simulink subsystem "battery_pack"  (R2021a)
settings: Solver=VariableStepAuto  StartTime=0.0  StopTime=10.0  RelTol=1e-3
values from neighbouring files (symbols this model uses):
  AmbientTemperature = 25 + 273.15    (= 298.15)    [battery_ws.m]
undefined symbols (not defined in the file or in its folder): BusbarRes, CellSeriesRes
libraries: fl_lib x11
settings Model: Creator=Carlo Edoardo  LastModifiedBy=Carlo Edoardo

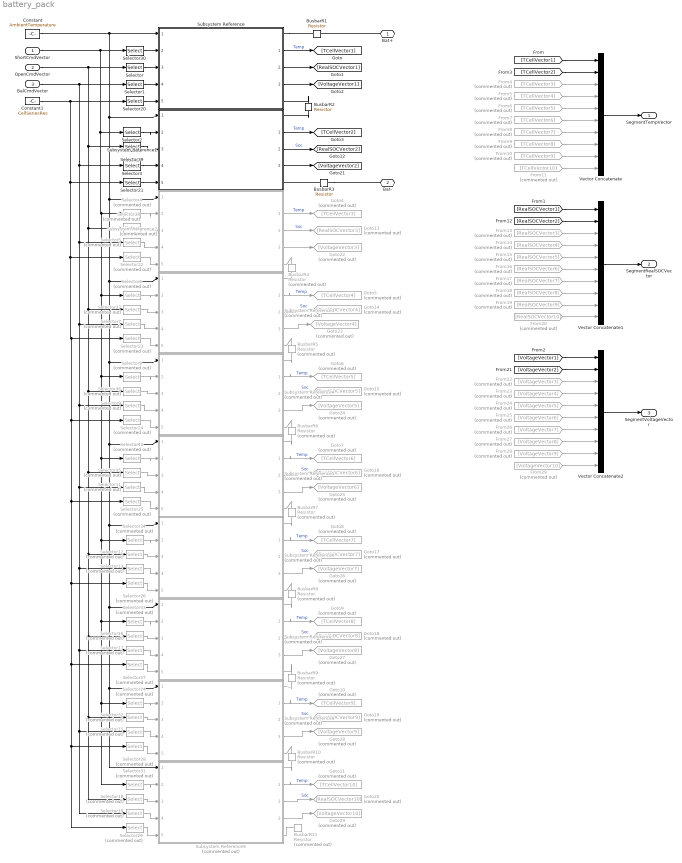
== system battery_pack ==
  ShortCmdVector : Inport
  OpenCmdVector : Inport  Port=2
  BalCmdVector : Inport  Port=3
  BusbarR1 : fl_lib/Electrical/Electrical Elements/Resistor  R=BusbarRes(1) Ohm  i_specify=off  i_priority=None  i=0 A  i_nominal_specify=off  i_nominal_unit=A  i_nominal_value=1  v_specify=off  v_priority=None  v=0 V  v_nominal_specify=off  v_nominal_unit=V  v_nominal_value=1
  BusbarR10 : fl_lib/Electrical/Electrical Elements/Resistor  Commented=on  R=BusbarRes(10) Ohm  i_specify=off  i_priority=None  i=0 A  i_nominal_specify=off  i_nominal_unit=A  i_nominal_value=1  v_specify=off  v_priority=None  v=0 V  v_nominal_specify=off  v_nominal_unit=V  v_nominal_value=1
  BusbarR11 : fl_lib/Electrical/Electrical Elements/Resistor  Commented=on  R=BusbarRes(11) Ohm  i_specify=off  i_priority=None  i=0 A  i_nominal_specify=off  i_nominal_unit=A  i_nominal_value=1  v_specify=off  v_priority=None  v=0 V  v_nominal_specify=off  v_nominal_unit=V  v_nominal_value=1
  BusbarR2 : fl_lib/Electrical/Electrical Elements/Resistor  R=BusbarRes(2) Ohm  i_specify=off  i_priority=None  i=0 A  i_nominal_specify=off  i_nominal_unit=A  i_nominal_value=1  v_specify=off  v_priority=None  v=0 V  v_nominal_specify=off  v_nominal_unit=V  v_nominal_value=1
  BusbarR3 : fl_lib/Electrical/Electrical Elements/Resistor  R=BusbarRes(3) Ohm  i_specify=off  i_priority=None  i=0 A  i_nominal_specify=off  i_nominal_unit=A  i_nominal_value=1  v_specify=off  v_priority=None  v=0 V  v_nominal_specify=off  v_nominal_unit=V  v_nominal_value=1
  BusbarR4 : fl_lib/Electrical/Electrical Elements/Resistor  Commented=on  R=BusbarRes(4) Ohm  i_specify=off  i_priority=None  i=0 A  i_nominal_specify=off  i_nominal_unit=A  i_nominal_value=1  v_specify=off  v_priority=None  v=0 V  v_nominal_specify=off  v_nominal_unit=V  v_nominal_value=1
  BusbarR5 : fl_lib/Electrical/Electrical Elements/Resistor  Commented=on  R=BusbarRes(5) Ohm  i_specify=off  i_priority=None  i=0 A  i_nominal_specify=off  i_nominal_unit=A  i_nominal_value=1  v_specify=off  v_priority=None  v=0 V  v_nominal_specify=off  v_nominal_unit=V  v_nominal_value=1
  BusbarR6 : fl_lib/Electrical/Electrical Elements/Resistor  Commented=on  R=BusbarRes(6) Ohm  i_specify=off  i_priority=None  i=0 A  i_nominal_specify=off  i_nominal_unit=A  i_nominal_value=1  v_specify=off  v_priority=None  v=0 V  v_nominal_specify=off  v_nominal_unit=V  v_nominal_value=1
  BusbarR7 : fl_lib/Electrical/Electrical Elements/Resistor  Commented=on  R=BusbarRes(7) Ohm  i_specify=off  i_priority=None  i=0 A  i_nominal_specify=off  i_nominal_unit=A  i_nominal_value=1  v_specify=off  v_priority=None  v=0 V  v_nominal_specify=off  v_nominal_unit=V  v_nominal_value=1
  BusbarR8 : fl_lib/Electrical/Electrical Elements/Resistor  Commented=on  R=BusbarRes(8) Ohm  i_specify=off  i_priority=None  i=0 A  i_nominal_specify=off  i_nominal_unit=A  i_nominal_value=1  v_specify=off  v_priority=None  v=0 V  v_nominal_specify=off  v_nominal_unit=V  v_nominal_value=1
  BusbarR9 : fl_lib/Electrical/Electrical Elements/Resistor  Commented=on  R=BusbarRes(9) Ohm  i_specify=off  i_priority=None  i=0 A  i_nominal_specify=off  i_nominal_unit=A  i_nominal_value=1  v_specify=off  v_priority=None  v=0 V  v_nominal_specify=off  v_nominal_unit=V  v_nominal_value=1
  Constant : Constant  Value=AmbientTemperature
  Constant1 : Constant  Value=CellSeriesRes
  From10 : From  Commented=on  GotoTag=TCellVector9
  From11 : From  Commented=on  GotoTag=TCellVector10
  From13 : From  Commented=on  GotoTag=RealSOCVector3
  From14 : From  Commented=on  GotoTag=RealSOCVector4
  From15 : From  Commented=on  GotoTag=RealSOCVector5
  From16 : From  Commented=on  GotoTag=RealSOCVector6
  From17 : From  Commented=on  GotoTag=RealSOCVector7
  From18 : From  Commented=on  GotoTag=RealSOCVector8
  From19 : From  Commented=on  GotoTag=RealSOCVector9
  From20 : From  Commented=on  GotoTag=RealSOCVector10
  From22 : From  Commented=on  GotoTag=VoltageVector3
  From23 : From  Commented=on  GotoTag=VoltageVector4
  From24 : From  Commented=on  GotoTag=VoltageVector5
  From25 : From  Commented=on  GotoTag=VoltageVector6
  From26 : From  Commented=on  GotoTag=VoltageVector7
  From27 : From  Commented=on  GotoTag=VoltageVector8
  From28 : From  Commented=on  GotoTag=VoltageVector9
  From29 : From  Commented=on  GotoTag=VoltageVector10
  From4 : From  Commented=on  GotoTag=TCellVector3
  From5 : From  Commented=on  GotoTag=TCellVector4
  From6 : From  Commented=on  GotoTag=TCellVector5
  From7 : From  Commented=on  GotoTag=TCellVector6
  From8 : From  Commented=on  GotoTag=TCellVector7
  From9 : From  Commented=on  GotoTag=TCellVector8
  Goto10 : Goto  Commented=on  GotoTag=TCellVector9
  Goto11 : Goto  Commented=on  GotoTag=TCellVector10
  Goto13 : Goto  Commented=on  GotoTag=RealSOCVector3
  Goto14 : Goto  Commented=on  GotoTag=RealSOCVector4
  Goto15 : Goto  Commented=on  GotoTag=RealSOCVector5
  Goto16 : Goto  Commented=on  GotoTag=RealSOCVector6
  Goto17 : Goto  Commented=on  GotoTag=RealSOCVector7
  Goto18 : Goto  Commented=on  GotoTag=RealSOCVector8
  Goto19 : Goto  Commented=on  GotoTag=RealSOCVector9
  Goto20 : Goto  Commented=on  GotoTag=RealSOCVector10
  Goto22 : Goto  Commented=on  GotoTag=VoltageVector3
  Goto23 : Goto  Commented=on  GotoTag=VoltageVector4
  Goto24 : Goto  Commented=on  GotoTag=VoltageVector5
  Goto25 : Goto  Commented=on  GotoTag=VoltageVector6
  Goto26 : Goto  Commented=on  GotoTag=VoltageVector7
  Goto27 : Goto  Commented=on  GotoTag=VoltageVector8
  Goto28 : Goto  Commented=on  GotoTag=VoltageVector9
  Goto29 : Goto  Commented=on  GotoTag=VoltageVector10
  Goto4 : Goto  Commented=on  GotoTag=TCellVector3
  Goto5 : Goto  Commented=on  GotoTag=TCellVector4
  Goto6 : Goto  Commented=on  GotoTag=TCellVector5
  Goto7 : Goto  Commented=on  GotoTag=TCellVector6
  Goto8 : Goto  Commented=on  GotoTag=TCellVector7
  Goto9 : Goto  Commented=on  GotoTag=TCellVector8
  Selector{,1,20,30} (4 alike) : Selector  InputPortWidth=10  IndexOptions=Index vector (dialog)  Indices=1  OutputSizes=1
  Selector{10..11,25,35} (4 alike) : Selector  Commented=on  InputPortWidth=10  IndexOptions=Index vector (dialog)  Indices=6  OutputSizes=1
  Selector{12..13,26,34} (4 alike) : Selector  Commented=on  InputPortWidth=10  IndexOptions=Index vector (dialog)  Indices=7  OutputSizes=1
  Selector{14..15,28,32} (4 alike) : Selector  Commented=on  InputPortWidth=10  IndexOptions=Index vector (dialog)  Indices=9  OutputSizes=1
  Selector{16..17,27,33} (4 alike) : Selector  Commented=on  InputPortWidth=10  IndexOptions=Index vector (dialog)  Indices=8  OutputSizes=1
  Selector{18..19,29,31} (4 alike) : Selector  Commented=on  InputPortWidth=10  IndexOptions=Index vector (dialog)  Indices=10  OutputSizes=1
  Selector{2..3,21,39} (4 alike) : Selector  InputPortWidth=10  IndexOptions=Index vector (dialog)  Indices=2  OutputSizes=1
  Selector{4..5,22,38} (4 alike) : Selector  Commented=on  InputPortWidth=10  IndexOptions=Index vector (dialog)  Indices=3  OutputSizes=1
  Selector{6..7,23,37} (4 alike) : Selector  Commented=on  InputPortWidth=10  IndexOptions=Index vector (dialog)  Indices=4  OutputSizes=1
  Selector{8..9,24,36} (4 alike) : Selector  Commented=on  InputPortWidth=10  IndexOptions=Index vector (dialog)  Indices=5  OutputSizes=1
  Subsystem Reference : Subsystem  ReferencedSubsystem=battery_module
      settings: PortSchema="{\"entries\":[{\"content\":{\"sides\":[{\"content\":{\"connectorIds\":[\"In1\",\"In2\",\"In3\",\"In4\",\"In5\"]},\"type\":\"ConnectorPlacement.EquallySpacedRectSide\",\"uuid\":\"f42d6b3d-39c7-468b-a9a7-4e5d796eba3b\"},{\"content\":{\"connectorIds\":[\"RConn1\",\"Out1\",\"Out2\",\"Out3\",\"RConn2\"],\"side\":\"RIGHT\"},\"type\":\"ConnectorPlacement.EquallySpacedRectSide\",\"uuid\":\"e762e236-7776-43b9-bd8d-fb7f2716d190\"},{\"content\":{\"connectorIds\":[],\"side\":\"TOP\"},\"type\":\"ConnectorPlacement.EquallySpacedRectSide\",\"uuid\":\"bd0c4b53-2dd2-497f-95b6-77c2ca394183\"}]},\"type\":\"ConnectorPlacement.EquallySpacedConnector\",\"uuid\":\"abacbee7-c859-4f21-9973-420371fecb92\"}],\"packageUris\":[\"http://schema.mathworks.com/mf0/Connector/R2020b\"],\"version\":\"1.0\"}"
  Subsystem Reference1 : Subsystem  ReferencedSubsystem=battery_module
      settings: PortSchema="{\"entries\":[{\"content\":{\"sides\":[{\"content\":{\"connectorIds\":[\"In1\",\"In2\",\"In3\",\"In4\",\"In5\"]},\"type\":\"ConnectorPlacement.EquallySpacedRectSide\",\"uuid\":\"f42d6b3d-39c7-468b-a9a7-4e5d796eba3b\"},{\"content\":{\"connectorIds\":[\"RConn1\",\"Out1\",\"Out2\",\"Out3\",\"RConn2\"],\"side\":\"RIGHT\"},\"type\":\"ConnectorPlacement.EquallySpacedRectSide\",\"uuid\":\"e762e236-7776-43b9-bd8d-fb7f2716d190\"},{\"content\":{\"connectorIds\":[],\"side\":\"TOP\"},\"type\":\"ConnectorPlacement.EquallySpacedRectSide\",\"uuid\":\"bd0c4b53-2dd2-497f-95b6-77c2ca394183\"}]},\"type\":\"ConnectorPlacement.EquallySpacedConnector\",\"uuid\":\"abacbee7-c859-4f21-9973-420371fecb92\"}],\"packageUris\":[\"http://schema.mathworks.com/mf0/Connector/R2020b\"],\"version\":\"1.0\"}"
  Subsystem Reference{2..9} (8 alike) : Subsystem  Commented=on  ReferencedSubsystem=battery_module
      settings: PortSchema="{\"entries\":[{\"content\":{\"sides\":[{\"content\":{\"connectorIds\":[\"In1\",\"In2\",\"In3\",\"In4\",\"In5\"]},\"type\":\"ConnectorPlacement.EquallySpacedRectSide\",\"uuid\":\"f42d6b3d-39c7-468b-a9a7-4e5d796eba3b\"},{\"content\":{\"connectorIds\":[\"RConn1\",\"Out1\",\"Out2\",\"Out3\",\"RConn2\"],\"side\":\"RIGHT\"},\"type\":\"ConnectorPlacement.EquallySpacedRectSide\",\"uuid\":\"e762e236-7776-43b9-bd8d-fb7f2716d190\"},{\"content\":{\"connectorIds\":[],\"side\":\"TOP\"},\"type\":\"ConnectorPlacement.EquallySpacedRectSide\",\"uuid\":\"bd0c4b53-2dd2-497f-95b6-77c2ca394183\"}]},\"type\":\"ConnectorPlacement.EquallySpacedConnector\",\"uuid\":\"abacbee7-c859-4f21-9973-420371fecb92\"}],\"packageUris\":[\"http://schema.mathworks.com/mf0/Connector/R2020b\"],\"version\":\"1.0\"}"
  Vector Concatenate : Concatenate  NumInputs=10
  Vector Concatenate1 : Concatenate  NumInputs=10
  Vector Concatenate2 : Concatenate  NumInputs=10
  Bat+ : PMIOPort  Side=Right
  Bat- : PMIOPort  Port=2  Side=Right
  SegmentTempVector : Outport
  SegmentRealSOCVector : Outport  Port=2
  SegmentVoltageVector : Outport  Port=3
  wires:
  Subsystem Reference8/1 -> Goto10/1  "Temp"
  [VoltageVector1] -> Vector Concatenate2/1
  Selector8/1 -> Subsystem Reference4/2
  Selector22/1 -> Subsystem Reference2/5
  Selector34/1 -> Subsystem Reference6/2
  From22/1 -> Vector Concatenate2/3
  Subsystem Reference8/2 -> Goto19/1  "Soc"
  From27/1 -> Vector Concatenate2/8
  Selector28/1 -> Subsystem Reference8/5
  ShortCmdVector/1 -> Selector30/1, Selector2/1, Selector4/1, Selector6/1, Selector8/1, Selector10/1, Selector34/1, Selector33/1, Selector14/1, Selector31/1
  Subsystem Reference5/2 -> Goto16/1  "Soc"
  Selector17/1 -> Subsystem Reference7/4
  From24/1 -> Vector Concatenate2/5
  Selector13/1 -> Subsystem Reference6/4
  From23/1 -> Vector Concatenate2/4
  From4/1 -> Vector Concatenate/3
  From16/1 -> Vector Concatenate1/6
  Selector6/1 -> Subsystem Reference3/2
  From5/1 -> Vector Concatenate/4
  Selector3/1 -> Subsystem Reference1/4
  From6/1 -> Vector Concatenate/5
  Constant/1 -> Subsystem Reference/1, Subsystem Reference3/1, Subsystem Reference9/1, Subsystem Reference8/1, Subsystem Reference7/1, Subsystem Reference6/1, Subsystem Reference5/1, Subsystem Reference4/1, Subsystem Reference2/1, Subsystem Reference1/1
  [VoltageVector2] -> Vector Concatenate2/2
  Subsystem Reference4/2 -> Goto15/1  "Soc"
  Selector25/1 -> Subsystem Reference5/5
  Selector10/1 -> Subsystem Reference5/2
  Selector35/1 -> Subsystem Reference5/3
  Subsystem Reference9/3 -> Goto29/1
  Subsystem Reference7/2 -> Goto18/1  "Soc"
  Selector24/1 -> Subsystem Reference4/5
  Constant1/1 -> Selector20/1, Selector21/1, Selector22/1, Selector23/1, Selector24/1, Selector25/1, Selector26/1, Selector27/1, Selector28/1, Selector29/1
  Selector37/1 -> Subsystem Reference3/3
  Subsystem Reference5/3 -> Goto25/1
  From29/1 -> Vector Concatenate2/10
  [TCellVector2] -> Vector Concatenate/2
  Subsystem Reference7/1 -> Goto9/1  "Temp"
  BalCmdVector/1 -> Selector1/1, Selector3/1, Selector5/1, Selector7/1, Selector9/1, Selector11/1, Selector13/1, Selector17/1, Selector15/1, Selector19/1
  From25/1 -> Vector Concatenate2/6
  From20/1 -> Vector Concatenate1/10
  Subsystem Reference6/3 -> Goto26/1
  Subsystem Reference4/1 -> Goto6/1  "Temp"
  From28/1 -> Vector Concatenate2/9
  Vector Concatenate2/1 -> SegmentVoltageVector/1
  Subsystem Reference3/1 -> Goto5/1  "Temp"
  Selector31/1 -> Subsystem Reference9/2
  From26/1 -> Vector Concatenate2/7
  Selector26/1 -> Subsystem Reference6/5
  Selector23/1 -> Subsystem Reference3/5
  Selector/1 -> Subsystem Reference/3
  Selector16/1 -> Subsystem Reference7/3
  Selector7/1 -> Subsystem Reference3/4
  From19/1 -> Vector Concatenate1/9
  Selector5/1 -> Subsystem Reference2/4
  Selector4/1 -> Subsystem Reference2/2
  Selector2/1 -> Subsystem Reference1/2
  Selector38/1 -> Subsystem Reference2/3
  Selector39/1 -> Subsystem Reference1/3
  From18/1 -> Vector Concatenate1/8
  Subsystem Reference3/2 -> Goto14/1  "Soc"
  Subsystem Reference/2 -> [RealSOCVector1]
  Subsystem Reference2/1 -> Goto4/1  "Temp"
  OpenCmdVector/1 -> Selector39/1, Selector38/1, Selector37/1, Selector36/1, Selector35/1, Selector12/1, Selector16/1, Selector32/1, Selector18/1, Selector/1
  Vector Concatenate1/1 -> SegmentRealSOCVector/1
  Subsystem Reference5/1 -> Goto7/1  "Temp"
  Subsystem Reference/1 -> [TCellVector1]  "Temp"
  [TCellVector1] -> Vector Concatenate/1
  From11/1 -> Vector Concatenate/10
  From8/1 -> Vector Concatenate/7
  Subsystem Reference/3 -> [VoltageVector1]
  Selector21/1 -> Subsystem Reference1/5
  From10/1 -> Vector Concatenate/9
  Subsystem Reference6/2 -> Goto17/1  "Soc"
  [RealSOCVector1] -> Vector Concatenate1/1
  Selector12/1 -> Subsystem Reference6/3
  From14/1 -> Vector Concatenate1/4
  From13/1 -> Vector Concatenate1/3
  Subsystem Reference2/2 -> Goto13/1  "Soc"
  Subsystem Reference9/2 -> Goto20/1  "Soc"
  Selector11/1 -> Subsystem Reference5/4
  Subsystem Reference1/2 -> [RealSOCVector2]  "Soc"
  From15/1 -> Vector Concatenate1/5
  Subsystem Reference2/3 -> Goto22/1
  From17/1 -> Vector Concatenate1/7
  Subsystem Reference4/3 -> Goto24/1
  From7/1 -> Vector Concatenate/6
  Subsystem Reference9/1 -> Goto11/1  "Temp"
  Subsystem Reference1/3 -> [VoltageVector2]
  Subsystem Reference3/3 -> Goto23/1
  Subsystem Reference1/1 -> [TCellVector2]  "Temp"
  Subsystem Reference6/1 -> Goto8/1  "Temp"
  [RealSOCVector2] -> Vector Concatenate1/2
  Selector1/1 -> Subsystem Reference/4
  Subsystem Reference7/3 -> Goto27/1
  From9/1 -> Vector Concatenate/8
  Vector Concatenate/1 -> SegmentTempVector/1
  Subsystem Reference8/3 -> Goto28/1
  Selector32/1 -> Subsystem Reference8/3
  Selector15/1 -> Subsystem Reference8/4
  Selector18/1 -> Subsystem Reference9/3
  Selector14/1 -> Subsystem Reference8/2
  Selector20/1 -> Subsystem Reference/5
  Selector19/1 -> Subsystem Reference9/4
  Selector30/1 -> Subsystem Reference/2
  Selector27/1 -> Subsystem Reference7/5
  Selector29/1 -> Subsystem Reference9/5
  Selector33/1 -> Subsystem Reference7/2
  Selector9/1 -> Subsystem Reference4/4
  Selector36/1 -> Subsystem Reference4/3
  connections:
  BusbarR4/LConn1 -- Subsystem Reference2/RConn2
  BusbarR6/LConn1 -- Subsystem Reference4/RConn2
  Subsystem Reference/RConn1 -- BusbarR1/RConn1
  BusbarR8/LConn1 -- Subsystem Reference6/RConn2
  BusbarR5/RConn1 -- Subsystem Reference4/RConn1
  BusbarR10/RConn1 -- Subsystem Reference9/RConn1
  BusbarR6/RConn1 -- Subsystem Reference5/RConn1
  BusbarR9/RConn1 -- Subsystem Reference8/RConn1
  BusbarR2/RConn1 -- Subsystem Reference1/RConn1
  BusbarR3/LConn1 -- Subsystem Reference1/RConn2
  BusbarR2/LConn1 -- Subsystem Reference/RConn2
  BusbarR5/LConn1 -- Subsystem Reference3/RConn2
  BusbarR7/RConn1 -- Subsystem Reference6/RConn1
  BusbarR7/LConn1 -- Subsystem Reference5/RConn2
  BusbarR8/RConn1 -- Subsystem Reference7/RConn1
  BusbarR11/RConn1 -- Subsystem Reference9/RConn2
  BusbarR4/RConn1 -- Subsystem Reference3/RConn1
  BusbarR9/LConn1 -- Subsystem Reference7/RConn2
  BusbarR10/LConn1 -- Subsystem Reference8/RConn2
  Bat+/RConn1 -- BusbarR1/LConn1
  BusbarR3/RConn1 -- Bat-/RConn1
